simulink model "rowstanu"  (R2013a)
settings: Solver=ode45  SolverMode=SingleTasking  StartTime=0.0  StopTime=20000  MaxStep=1  RelTol=1e-3
values from neighbouring files (symbols this model uses):
  A = [(-1*(Kg+cpp*rop*Fg0))/(Cvg) (Kg+cpp*rop*Fg0)/(Cvg); (Kg+cpp*rop*Fg0)/(Cvw) (-1*(Kg+K1+cpp*rop*Fg0))/(Cvw)]    [skrypt.m]
  B = [0 1/Cvg; K1/Cvw 0]    [skrypt.m]
  C = eye(2)    [skrypt.m]
  D = zeros(2)    [skrypt.m]
  dQg = 0    [skrypt.m]
  dTzew = 0    [skrypt.m]
  Qg0 = QgN    (= 20000)    [skrypt.m]
  t0 = 5000    [skrypt.m]
  Tzew0 = TzewN    (= -20)    [skrypt.m]
  x0 = ((-A)^(-1))*B*u0    [skrypt.m]
settings Model: Creator=LAB320-1552  LastModifiedBy=LAB320-1552
settings DataIOCC: SignalLoggingSaveFormat=ModelDataLogs
settings OptimizationCC: BlockReduction=off  BooleanDataType=off
settings DebuggingCC: SaveWithParameterizedLinksMsg=none  SignalResolutionControl=TryResolveAllWithWarning  SolverPrmCheckMsg=none  MultiTaskDSMMsg=warning  MultiTaskCondExecSysMsg=none  StrictBusMsg=None
settings HardwareCC: TargetUnknown=on
settings RTWCC: IncludeERTFirstTime=on

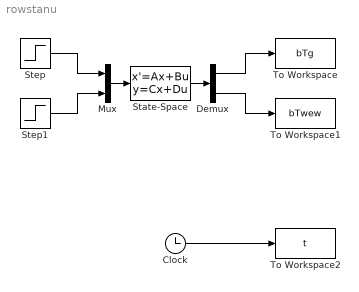
== system rowstanu ==
  Clock : Clock
  Demux : Demux  Outputs=2
  Mux : Mux  Inputs=2
  State-Space : StateSpace  A=A  B=B  C=C  D=D  X0=x0
  Step : Step  Time=t0  Before=Tzew0  After=Tzew0+dTzew  SampleTime=0
  Step1 : Step  Time=t0  Before=Qg0  After=Qg0+dQg  SampleTime=0
  To Workspace : ToWorkspace  VariableName=bTg  SampleTime=-1
  To Workspace1 : ToWorkspace  VariableName=bTwew  SampleTime=-1
  To Workspace2 : ToWorkspace  VariableName=t  SampleTime=-1
  wires:
  Mux/1 -> State-Space/1
  State-Space/1 -> Demux/1
  Demux/1 -> To Workspace/1
  Demux/2 -> To Workspace1/1
  Step/1 -> Mux/1
  Step1/1 -> Mux/2
  Clock/1 -> To Workspace2/1
